simulink model "TiltExp_v3"  (R2016a)
settings: Solver=ode4  StartTime=0.0  StopTime=Inf  FixedStep=1/sr_stim  RelTol=1e-3
StopFcn:
  | stopSimulation
model workspace (MAT data in the model file):
  simTime = 10
  sr = 1000
  sr_stim = 1000
undefined symbols (not defined in the file): DiscIntNeverNeededParam, NCh_select
libraries: xpcutilitieslib x8, slrtlib x6, speedgoatlib_IO102 x3, dspsigops x3, simulink_extras x2, simulink x1
settings Model: SimulationMode=external  Creator=PosturalControlLab  LastModifiedBy=PosturalControlLab
settings SolverCC: EnableConcurrentExecution=on
settings DataIOCC: ExternalInput=data  SaveFormat=StructureWithTime  SaveOutput=off  SignalLogging=off  DSMLogging=off  SaveTime=off
settings OptimizationCC: BlockReduction=off  OptimizeBlockIOStorage=off  BufferReuse=off  GlobalBufferReuse=off  ExpressionFolding=off  LocalBlockOutputs=off
settings HardwareCC: ProdBitPerPointer=32  ProdLargestAtomicFloat=None  ProdWordSize=32  ProdLongLongMode=on  ProdHWDeviceType=Generic->32-bit x86 compatible
settings RTWCC: SystemTargetFile=slrt.tlc  TemplateMakefile=slrt_default_tmf  Description=Simulink Real-Time  RTWCompilerOptimization=on

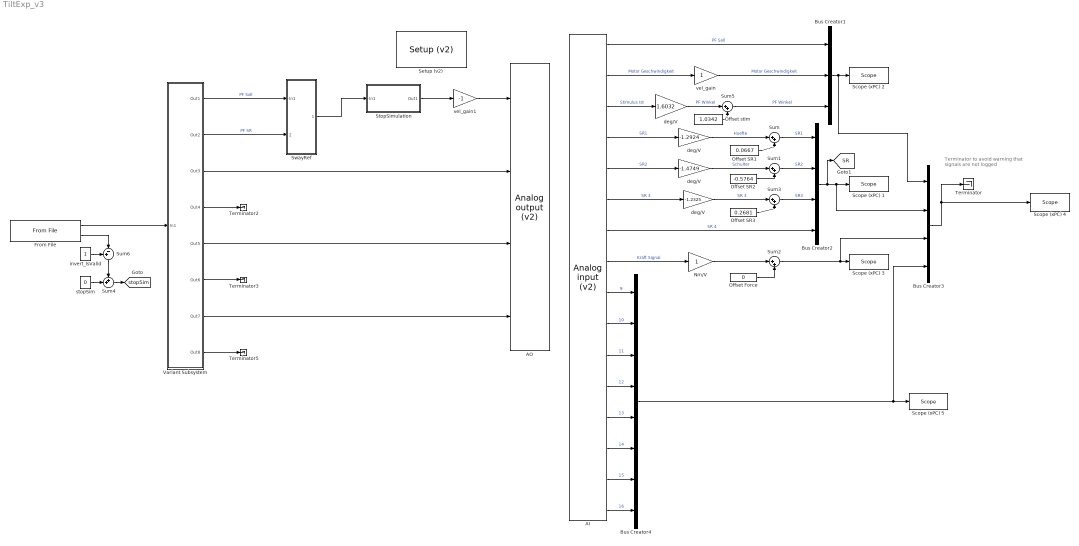
== system TiltExp_v3 ==
  note: Terminator to avoid warning
      | that signals are not logged
  AI : speedgoatlib_IO102/Analog input (v2)   id=1  channels=[1 2 3 4 5 6 7 8 9 10 11 12 13 14 15 16]  range=1  high_voltage=off  adCoupling=2  ts=1/sr  pciSlot=-1
  "AO " : speedgoatlib_IO102/Analog output (v2)   id=1  channels=[1 2 3 4]  range=1  ts=1/sr  pciSlot=-1
  Bus Creator1 : BusCreator  Inputs=3
  Bus Creator2 : BusCreator  Inputs=4
  Bus Creator3 : BusCreator  Inputs=4
  Bus Creator4 : BusCreator  Inputs=8
  "From File " : slrtlib/Target Management/From File   filename='stim.dat'  dataSize=NCh_select*8  bufSize=102400  readSize=1024  EOFOption=Hold last output  sampTime=1/sr_stim  show2ports=on
  Nm/V : Gain
  Offset Force : Constant  Value=0
  Offset SR1 : Constant  Value=0.0667
  Offset SR2 : Constant  Value=-0.5764
  Offset SR3 : Constant  Value=0.2681
  Offset stim : Constant  Value=1.0342
  Scope (xPC) 1 : slrtlib/Displays and Logging/Scope   scopeno=2  scopetype=Target  autostart=on  viewmode=Graphical sliding  formatstr='%15.6f'  grid=on  ylimits=[-10,10]  nosamples=10000  noprepostsamples=0  interleave=20  triggermode=FreeRun  triggersignal=1  trigsignalfromport=off  triggerlevel=0.0  triggerslope=Rising  triggerscope=1  triggersample=0  filename=data.dat  mode=Lazy  writesize=512  autorestart=off  dynamicfilemode=off  maxwritefilesize=512*1024^2
  Scope (xPC) 2 : slrtlib/Displays and Logging/Scope   scopeno=1  scopetype=Target  autostart=on  viewmode=Graphical sliding  formatstr='%15.6f'  grid=on  ylimits=[-5,5]  nosamples=10000  noprepostsamples=0  interleave=20  triggermode=FreeRun  triggersignal=1  trigsignalfromport=off  triggerlevel=0.0  triggerslope=Rising  triggerscope=1  triggersample=0  filename=data.dat  mode=Lazy  writesize=512  autorestart=off  dynamicfilemode=off  maxwritefilesize=512*1024^2
  Scope (xPC) 3 : slrtlib/Displays and Logging/Scope   scopeno=3  scopetype=Target  autostart=on  viewmode=Graphical sliding  formatstr='%15.6f'  grid=on  ylimits=[-5,5]  nosamples=10000  noprepostsamples=0  interleave=20  triggermode=FreeRun  triggersignal=1  trigsignalfromport=off  triggerlevel=0.0  triggerslope=Rising  triggerscope=1  triggersample=0  filename=data.dat  mode=Lazy  writesize=512  autorestart=off  dynamicfilemode=off  maxwritefilesize=512*1024^2
  Scope (xPC) 4 : slrtlib/Displays and Logging/Scope   scopeno=5  scopetype=File  autostart=on  viewmode=Graphical sliding  formatstr='%15.6f'  grid=on  ylimits=[-5,5]  nosamples=10000  noprepostsamples=0  interleave=1  triggermode=FreeRun  triggersignal=1  trigsignalfromport=on  triggerlevel=1  triggerslope=Rising  triggerscope=1  triggersample=0  filename=data.dat  mode=Lazy  writesize=2048  autorestart=off  dynamicfilemode=off  maxwritefilesize=512*1024^2
  Scope (xPC) 5 : slrtlib/Displays and Logging/Scope   scopeno=4  scopetype=Target  autostart=on  viewmode=Graphical sliding  formatstr='%15.6f'  grid=on  ylimits=[-5,5]  nosamples=10000  noprepostsamples=0  interleave=20  triggermode=FreeRun  triggersignal=1  trigsignalfromport=off  triggerlevel=0.0  triggerslope=Rising  triggerscope=1  triggersample=0  filename=data.dat  mode=Lazy  writesize=512  autorestart=off  dynamicfilemode=off  maxwritefilesize=512*1024^2
  "Setup (v2) " : speedgoatlib_IO102/Setup (v2)   id=1  range=+-10V  cal=off  pciSlot=-1  adCoupling=Single-ended  adChannelMode=Multiple-channel (enter number of channels below)  adChannel=16  daChannel=[1,2,3,4]  daReset=[1]  daInitValue=[0]  DioDirectionLo=Input  DioDirectionHi=Output  doChannel=[9]  doReset=[1]  doInitValue=[0]  diChannel=[1]
  StopSimulation : Subsystem
  Sum{,1..3,5} (5 alike) : Sum  Inputs=|++
  Sum4 : Sum  Inputs=++|
  Sum6 : Sum  Inputs=+-|
  SwayRef : Subsystem
  Terminator{,2..3,5} (4 alike) : Terminator
  Variant Subsystem : Subsystem  Variant=on
  deg/V : Gain  Gain=1.6032
  "deg/V " : Gain  Gain=-1.2924
  "deg/V  " : Gain  Gain=-1.4749
  "deg/V   " : Gain  Gain=-1.2325
  invert_IsValid : Constant
  stopSim : Constant  Value=0
  vel_gain : Gain
  vel_gain1 : Gain  Gain=-1
  tag scope: SR=global, stopSim=global
  wires:
  AI/1 -> Bus Creator1/1  "PF Soll"
  AI/3 -> deg/V/1  "Stimulus Ist"
  AI/2 -> vel_gain/1  "Motor Geschwindigkeit"
  Bus Creator1/1 -> Bus Creator3/1, Scope (xPC) 2/1
  AI/8 -> Nm/V/1  "Kraft Signal"
  "From File "/1 -> Variant Subsystem/1(In1)
  Sum5/1 -> Bus Creator1/3  "PF Winkel"
  Offset SR1/1 -> Sum/2
  Offset SR2/1 -> Sum1/2
  Offset SR3/1 -> Sum3/2
  Bus Creator2/1 -> [SR], Bus Creator3/2, Scope (xPC) 1/1
  "deg/V "/1 -> Sum/1  "Huefte"
  "deg/V  "/1 -> Sum1/1  "Schulter"
  "deg/V   "/1 -> Sum3/1  "SR 3"
  AI/7 -> Bus Creator2/4  "SR 4"
  Sum3/1 -> Bus Creator2/3  "SR3"
  Sum1/1 -> Bus Creator2/2  "SR2"
  Sum/1 -> Bus Creator2/1  "SR1"
  AI/4 -> "deg/V "/1  "SR1"
  AI/5 -> "deg/V  "/1  "SR2"
  AI/6 -> "deg/V   "/1  "SR 3"
  Bus Creator3/1 -> Scope (xPC) 4/1, Terminator/1
  Variant Subsystem/4(Out4) -> Terminator2/1
  Variant Subsystem/5(Out5) -> "AO "/3
  Variant Subsystem/6(Out6) -> Terminator3/1
  Variant Subsystem/7(Out7) -> "AO "/4
  Variant Subsystem/8(Out8) -> Terminator5/1
  AI/15 -> Bus Creator4/7  "15"
  AI/16 -> Bus Creator4/8  "16"
  AI/14 -> Bus Creator4/6  "14"
  AI/13 -> Bus Creator4/5  "13"
  AI/11 -> Bus Creator4/3  "11"
  AI/12 -> Bus Creator4/4  "12"
  AI/10 -> Bus Creator4/2  "10"
  AI/9 -> Bus Creator4/1  "9"
  Bus Creator4/1 -> Scope (xPC) 5/1, Bus Creator3/4
  Variant Subsystem/1(Out1) -> SwayRef/1(In1)  "PF Soll"
  Variant Subsystem/2(Out2) -> SwayRef/2(SR on/off)  "PF SR"
  SwayRef/1(Out1) -> StopSimulation/1(In1)
  stopSim/1 -> Sum4/2
  Variant Subsystem/3(Out3) -> "AO "/2
  StopSimulation/1(Out1) -> vel_gain1/1
  vel_gain/1 -> Bus Creator1/2  "Motor Geschwindigkeit"
  Offset stim/1 -> Sum5/2
  Sum2/1 -> Bus Creator3/3, Scope (xPC) 3/1
  Nm/V/1 -> Sum2/1
  Offset Force/1 -> Sum2/2
  "From File "/2 -> Sum6/2
  Sum4/1 -> [stopSim]
  invert_IsValid/1 -> Sum6/1
  Sum6/1 -> Sum4/1
  deg/V/1 -> Sum5/1  "PF Winkel"
  vel_gain1/1 -> "AO "/1

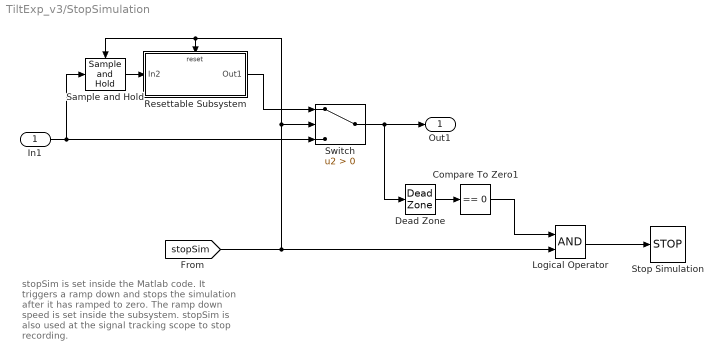
== system TiltExp_v3/StopSimulation ==
  note: stopSim is set inside the Matlab code.
      | It triggers a ramp down and stops the
      | simulation after it has ramped to zero.
      | The ramp down speed is set inside the
      | subsystem.
      |
      | stopSim is also used at the signal tracking
      | scope to stop recording.
  In1 : Inport
  Compare To Zero1 : simulink/Logic and Bit Operations/Compare To Zero  relop===  OutDataTypeStr=boolean
  Dead Zone : DeadZone  LowerValue=-0.01  UpperValue=0.01  SaturateOnIntegerOverflow=on
  Logical Operator : Logic  AllPortsSameDT=off  OutDataTypeStr=boolean
  Resettable Subsystem : Subsystem  TreatAsAtomicUnit=on
  Sample and Hold : dspsigops/Sample and Hold  trig=Either edge  initCond=0  latchinput=off
  Stop Simulation : Stop
  Switch : Switch  Criteria=u2 > Threshold
  Out1 : Outport
  wires:
  [stopSim] -> Sample and Hold/Trigger, Resettable Subsystem/Reset, Switch/2, Logical Operator/2
  Resettable Subsystem/1(Out1) -> Switch/1
  In1/1 -> Sample and Hold/1, Switch/3
  Logical Operator/1 -> Stop Simulation/1
  Switch/1 -> Out1/1, Dead Zone/1
  Sample and Hold/1 -> Resettable Subsystem/1(In2)
  Compare To Zero1/1 -> Logical Operator/1
  Dead Zone/1 -> Compare To Zero1/1

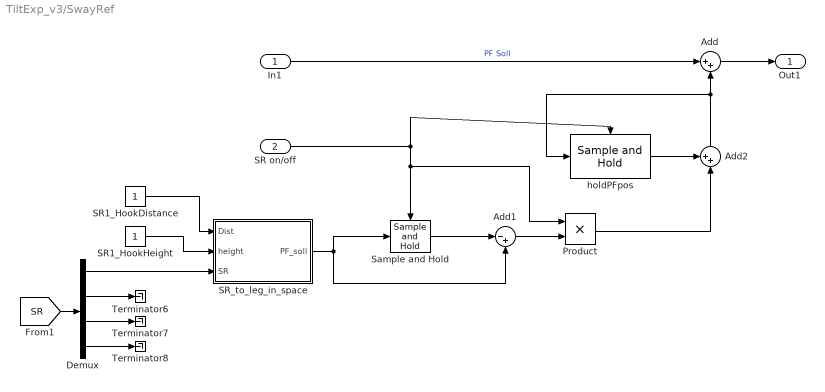
== system TiltExp_v3/SwayRef ==
  In1 : Inport
  SR on/off : Inport  Port=2
  Add : Sum  Inputs=|++
  Add1 : Sum  Inputs=|-+
  Add2 : Sum  Inputs=++|
  Demux : Demux
  Product : Product
  SR1_HookDistance : Constant
  SR1_HookHeight : Constant
  SR_to_leg_in_space : Subsystem
  Sample and Hold : dspsigops/Sample and Hold  trig=Rising edge  initCond=0  latchinput=off
  Terminator6 : Terminator
  Terminator7 : Terminator
  Terminator8 : Terminator
  holdPFpos : dspsigops/Sample and Hold  RequirementInfo="{}  %GIDa_cbccdeba_99ff_497b_8873_f2096e792c9e"  trig=Falling edge  initCond=0  latchinput=on
  Out1 : Outport
  wires:
  Demux/2 -> Terminator6/1
  Demux/3 -> Terminator7/1
  Demux/4 -> Terminator8/1
  [SR] -> Demux/1
  SR1_HookDistance/1 -> SR_to_leg_in_space/1("Dist ")
  SR1_HookHeight/1 -> SR_to_leg_in_space/2("height ")
  Demux/1 -> SR_to_leg_in_space/3(SR)
  Add/1 -> Out1/1
  In1/1 -> Add/1  "PF Soll"
  SR on/off/1 -> holdPFpos/Trigger, Product/1, Sample and Hold/Trigger
  SR_to_leg_in_space/1(PF_soll) -> Add1/2, Sample and Hold/1
  Sample and Hold/1 -> Add1/1
  Add1/1 -> Product/2
  Product/1 -> Add2/2
  Add2/1 -> holdPFpos/1, Add/2
  holdPFpos/1 -> Add2/1

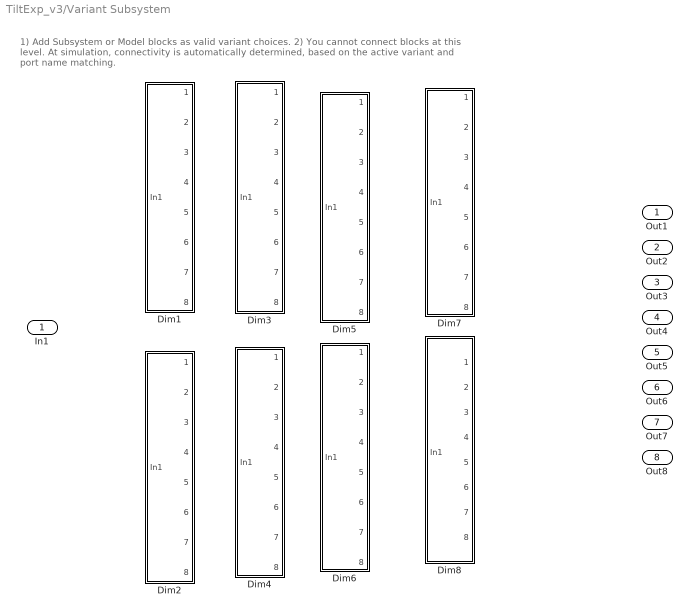
== system TiltExp_v3/Variant Subsystem ==
  note: 1) Add Subsystem or Model blocks as valid variant choices.
      | 2) You cannot connect blocks at this level. At simulation, connectivity is automatically
      | determined, based on the active variant and port name matching.
  In1 : Inport
  Dim1 : Subsystem  VariantControl=Var_NCh_1
  Dim2 : Subsystem  VariantControl=Var_NCh_2
  Dim3 : Subsystem  VariantControl=Var_NCh_3
  Dim4 : Subsystem  VariantControl=Var_NCh_4
  Dim5 : Subsystem  VariantControl=Var_NCh_5
  Dim6 : Subsystem  VariantControl=Var_NCh_6
  Dim7 : Subsystem  VariantControl=Var_NCh_7
  Dim8 : Subsystem  VariantControl=Var_NCh_8
  Out1 : Outport
  Out2 : Outport  Port=2
  Out3 : Outport  Port=3
  Out4 : Outport  Port=4
  Out5 : Outport  Port=5
  Out6 : Outport  Port=6
  Out7 : Outport  Port=7
  Out8 : Outport  Port=8

== system TiltExp_v3/StopSimulation/Resettable Subsystem ==
  In2 : Inport
  Reset : ResetPort  DisableCoverage=on
  Add : Sum  Inputs=|++
  Discrete-Time Integrator : DiscreteIntegrator  InitialConditionSetting=State (most efficient)  SampleTime=-1  ICPrevOutput=DiscIntNeverNeededParam  ICPrevScaledInput=DiscIntNeverNeededParam
  Product : Product
  Sign : Signum
  rampVelocity : Constant  Value=-2
  Out1 : Outport
  wires:
  rampVelocity/1 -> Discrete-Time Integrator/1
  Discrete-Time Integrator/1 -> Product/1
  Add/1 -> Out1/1
  In2/1 -> Add/2, Sign/1
  Sign/1 -> Product/2
  Product/1 -> Add/1

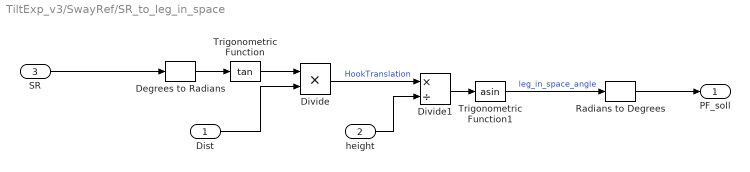
== system TiltExp_v3/SwayRef/SR_to_leg_in_space ==
  "Dist " : Inport
  "height " : Inport  Port=2
  SR : Inport  Port=3
  Degrees to Radians : simulink_extras/Transformations/Degrees to Radians
  Divide : Product  Inputs=**
  Divide1 : Product  Inputs=*/
  Radians to Degrees : simulink_extras/Transformations/Radians to Degrees
  Trigonometric Function : Trigonometry  Operator=tan
  Trigonometric Function1 : Trigonometry  Operator=asin
  PF_soll : Outport
  wires:
  Divide/1 -> Divide1/1  "HookTranslation"
  SR/1 -> Degrees to Radians/1
  "Dist "/1 -> Divide/2
  Trigonometric Function/1 -> Divide/1
  Radians to Degrees/1 -> PF_soll/1
  Divide1/1 -> Trigonometric Function1/1
  Trigonometric Function1/1 -> Radians to Degrees/1  "leg_in_space_angle"
  "height "/1 -> Divide1/2
  Degrees to Radians/1 -> Trigonometric Function/1

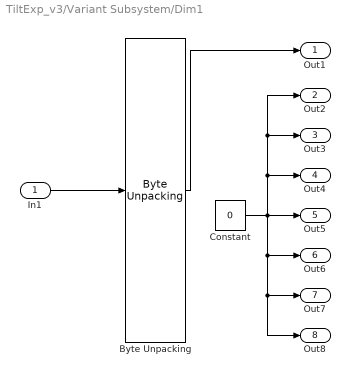
== system TiltExp_v3/Variant Subsystem/Dim1 ==
  In1 : Inport
  "Byte Unpacking " : xpcutilitieslib/Byte Unpacking   MaskUnpackedDataTypes={'double'}  MaskUnpackedDataSizes={[1]}  MaskAlignment=1
  Constant : Constant  Value=0
  Out1 : Outport
  Out2 : Outport  Port=2
  Out3 : Outport  Port=3
  Out4 : Outport  Port=4
  Out5 : Outport  Port=5
  Out6 : Outport  Port=6
  Out7 : Outport  Port=7
  Out8 : Outport  Port=8
  wires:
  Constant/1 -> Out8/1, Out7/1, Out6/1, Out2/1, Out3/1, Out4/1, Out5/1
  "Byte Unpacking "/1 -> Out1/1
  In1/1 -> "Byte Unpacking "/1

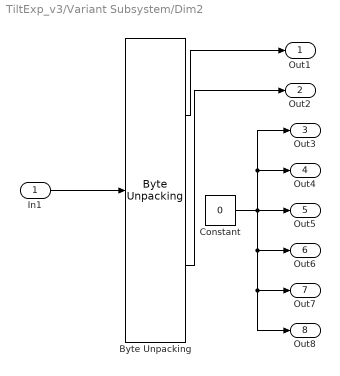
== system TiltExp_v3/Variant Subsystem/Dim2 ==
  In1 : Inport
  "Byte Unpacking " : xpcutilitieslib/Byte Unpacking   MaskUnpackedDataTypes={'double','double'}  MaskUnpackedDataSizes={[1], [1]}  MaskAlignment=1
  Constant : Constant  Value=0
  Out1 : Outport
  Out2 : Outport  Port=2
  Out3 : Outport  Port=3
  Out4 : Outport  Port=4
  Out5 : Outport  Port=5
  Out6 : Outport  Port=6
  Out7 : Outport  Port=7
  Out8 : Outport  Port=8
  wires:
  "Byte Unpacking "/2 -> Out2/1
  "Byte Unpacking "/1 -> Out1/1
  In1/1 -> "Byte Unpacking "/1
  Constant/1 -> Out8/1, Out7/1, Out6/1, Out3/1, Out4/1, Out5/1

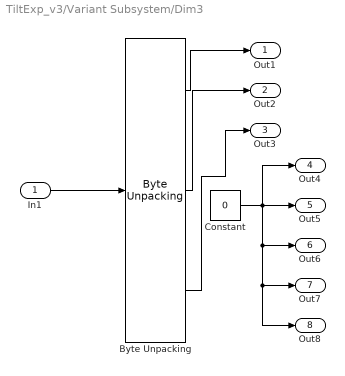
== system TiltExp_v3/Variant Subsystem/Dim3 ==
  In1 : Inport
  "Byte Unpacking " : xpcutilitieslib/Byte Unpacking   MaskUnpackedDataTypes={'double','double','double'}  MaskUnpackedDataSizes={[1], [1], [1]}  MaskAlignment=1
  Constant : Constant  Value=0
  Out1 : Outport
  Out2 : Outport  Port=2
  Out3 : Outport  Port=3
  Out4 : Outport  Port=4
  Out5 : Outport  Port=5
  Out6 : Outport  Port=6
  Out7 : Outport  Port=7
  Out8 : Outport  Port=8
  wires:
  "Byte Unpacking "/3 -> Out3/1
  "Byte Unpacking "/2 -> Out2/1
  "Byte Unpacking "/1 -> Out1/1
  In1/1 -> "Byte Unpacking "/1
  Constant/1 -> Out8/1, Out7/1, Out6/1, Out4/1, Out5/1

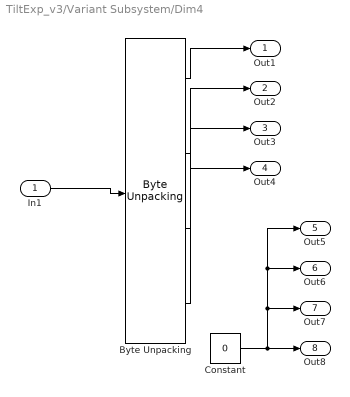
== system TiltExp_v3/Variant Subsystem/Dim4 ==
  In1 : Inport
  "Byte Unpacking " : xpcutilitieslib/Byte Unpacking   MaskUnpackedDataTypes={'double','double','double','double'}  MaskUnpackedDataSizes={[1], [1], [1], [1]}  MaskAlignment=1
  Constant : Constant  Value=0
  Out1 : Outport
  Out2 : Outport  Port=2
  Out3 : Outport  Port=3
  Out4 : Outport  Port=4
  Out5 : Outport  Port=5
  Out6 : Outport  Port=6
  Out7 : Outport  Port=7
  Out8 : Outport  Port=8
  wires:
  "Byte Unpacking "/4 -> Out4/1
  "Byte Unpacking "/3 -> Out3/1
  "Byte Unpacking "/2 -> Out2/1
  "Byte Unpacking "/1 -> Out1/1
  In1/1 -> "Byte Unpacking "/1
  Constant/1 -> Out5/1, Out6/1, Out7/1, Out8/1

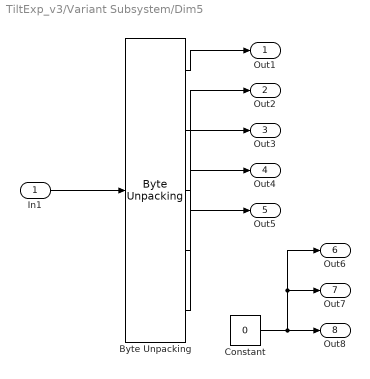
== system TiltExp_v3/Variant Subsystem/Dim5 ==
  In1 : Inport
  "Byte Unpacking " : xpcutilitieslib/Byte Unpacking   MaskUnpackedDataTypes={'double','double','double','double','double'}  MaskUnpackedDataSizes={[1], [1], [1], [1],[1]}  MaskAlignment=1
  Constant : Constant  Value=0
  Out1 : Outport
  Out2 : Outport  Port=2
  Out3 : Outport  Port=3
  Out4 : Outport  Port=4
  Out5 : Outport  Port=5
  Out6 : Outport  Port=6
  Out7 : Outport  Port=7
  Out8 : Outport  Port=8
  wires:
  "Byte Unpacking "/5 -> Out5/1
  "Byte Unpacking "/4 -> Out4/1
  "Byte Unpacking "/3 -> Out3/1
  "Byte Unpacking "/2 -> Out2/1
  "Byte Unpacking "/1 -> Out1/1
  In1/1 -> "Byte Unpacking "/1
  Constant/1 -> Out6/1, Out7/1, Out8/1

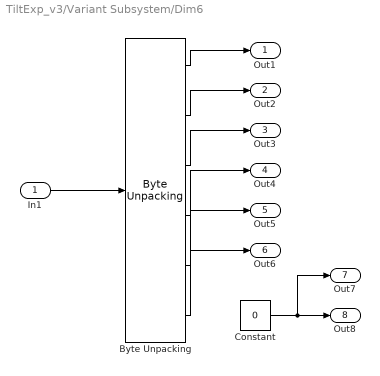
== system TiltExp_v3/Variant Subsystem/Dim6 ==
  In1 : Inport
  "Byte Unpacking " : xpcutilitieslib/Byte Unpacking   MaskUnpackedDataTypes={'double','double','double','double','double','double'}  MaskUnpackedDataSizes={[1], [1], [1], [1],[1], [1]}  MaskAlignment=1
  Constant : Constant  Value=0
  Out1 : Outport
  Out2 : Outport  Port=2
  Out3 : Outport  Port=3
  Out4 : Outport  Port=4
  Out5 : Outport  Port=5
  Out6 : Outport  Port=6
  Out7 : Outport  Port=7
  Out8 : Outport  Port=8
  wires:
  "Byte Unpacking "/6 -> Out6/1
  "Byte Unpacking "/5 -> Out5/1
  "Byte Unpacking "/4 -> Out4/1
  "Byte Unpacking "/3 -> Out3/1
  "Byte Unpacking "/2 -> Out2/1
  "Byte Unpacking "/1 -> Out1/1
  In1/1 -> "Byte Unpacking "/1
  Constant/1 -> Out7/1, Out8/1

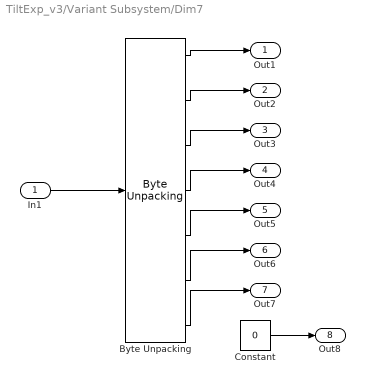
== system TiltExp_v3/Variant Subsystem/Dim7 ==
  In1 : Inport
  "Byte Unpacking " : xpcutilitieslib/Byte Unpacking   MaskUnpackedDataTypes={'double','double','double','double','double','double','double'}  MaskUnpackedDataSizes={[1], [1], [1], [1],[1], [1], [1]}  MaskAlignment=1
  Constant : Constant  Value=0
  Out1 : Outport
  Out2 : Outport  Port=2
  Out3 : Outport  Port=3
  Out4 : Outport  Port=4
  Out5 : Outport  Port=5
  Out6 : Outport  Port=6
  Out7 : Outport  Port=7
  Out8 : Outport  Port=8
  wires:
  "Byte Unpacking "/7 -> Out7/1
  "Byte Unpacking "/6 -> Out6/1
  "Byte Unpacking "/5 -> Out5/1
  "Byte Unpacking "/4 -> Out4/1
  "Byte Unpacking "/3 -> Out3/1
  "Byte Unpacking "/2 -> Out2/1
  "Byte Unpacking "/1 -> Out1/1
  In1/1 -> "Byte Unpacking "/1
  Constant/1 -> Out8/1

== system TiltExp_v3/Variant Subsystem/Dim8 ==
  In1 : Inport
  "Byte Unpacking " : xpcutilitieslib/Byte Unpacking   MaskUnpackedDataTypes={'double','double','double','double','double','double','double','double'}  MaskUnpackedDataSizes={[1], [1], [1], [1],[1], [1], [1], [1]}  MaskAlignment=1
  Out1 : Outport
  Out2 : Outport  Port=2
  Out3 : Outport  Port=3
  Out4 : Outport  Port=4
  Out5 : Outport  Port=5
  Out6 : Outport  Port=6
  Out7 : Outport  Port=7
  Out8 : Outport  Port=8
  wires:
  "Byte Unpacking "/7 -> Out7/1
  "Byte Unpacking "/8 -> Out8/1
  "Byte Unpacking "/6 -> Out6/1
  "Byte Unpacking "/5 -> Out5/1
  "Byte Unpacking "/4 -> Out4/1
  "Byte Unpacking "/3 -> Out3/1
  "Byte Unpacking "/2 -> Out2/1
  "Byte Unpacking "/1 -> Out1/1
  In1/1 -> "Byte Unpacking "/1
